simulink model "STEP2_W"  (Simulink 8.6)
settings: Solver=ode4  SolverMode=SingleTasking  StartTime=0.0  StopTime=inf  FixedStep=2/64e5  RelTol=1e-3
undefined symbols (not defined in the file or in its folder): get
libraries: system_blocks x3, measurement_tools x2, dspsnks4 x1
settings Model: MAModelExclusionFileProxy=C:\Users\user\Desktop\HAW\Digital Communication Systems\labs\Matlab\STEP2_W_exclusions.xml  Creator=Schoenen  LastModifiedBy=user
settings DataIOCC: SaveOutput=off  SaveTime=off  SignalLoggingName=sigsOut
settings OptimizationCC: BooleanDataType=off  ExpressionDepthLimit=128
settings DebuggingCC: SaveWithParameterizedLinksMsg=none  SignalResolutionControl=TryResolveAllWithWarning  SolverPrmCheckMsg=none  MultiTaskDSMMsg=warning  MultiTaskCondExecSysMsg=none  FcnCallInpInsideContextMsg=EnableAllAsError  StateNameClashWarn=none
settings HardwareCC: TargetUnknown=on
settings CodeAppCC: IgnoreCustomStorageClasses=off
settings ConfigComp: CovSFcnEnable=off

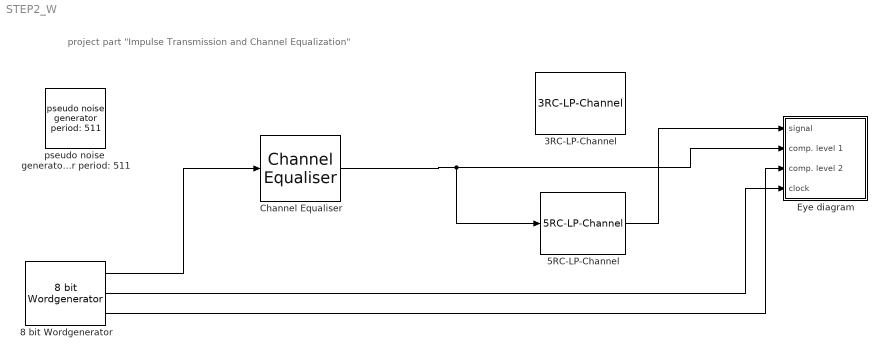
== system STEP2_W ==
  note: project part "Impulse Transmission and Channel Equalization"
  "3RC-LP-Channel " : system_blocks/3RC-LP-Channel   noise=0.1  a=off  step=2/64e5
  "5RC-LP-Channel " : system_blocks/5RC-LP-Channel   noise=0.1  a=off  step=2/64e5
  8 bit Wordgenerator : measurement_tools/8 bit Wordgenerator  word=[1 0 0 0 0 0 0 0]  bt=64000
  Channel Equaliser : system_blocks/Channel Equaliser
      link override c1: low=-1  gain=-0.733  high=1
      link override c2: low=-1  gain=0.227  high=1
      link override c3: low=-1  gain=-0.049  high=1
      link override c4: low=-1  gain=0.0026  high=1
  Eye diagram : Subsystem  AncestorBlock=measurement_tools/Eye diagram  mask{Tsymb=1, Tfss=2/64e5, ns=4, ndisplay=1, ymin=-2, ymax=2}
      mask prompts: Tsymb "symbol period [s]:"; Tfss "simulation step size [s]:"; ns "symbols per eye diagram (min. 4xndisplay):"; ndisplay "display time scale [ndisplay=number of symbols]:"
      mask init:
      | SampPerSymb = round(Tsymb/Tfss);
      | nsymb=ndisplay*ceil(ns/ndisplay);
  pseudo noise  generator period: 511 : measurement_tools/pseudo noise  generator period: 511  Tsymb=1  pol=unipolar  Tfss=2/64e5
  wires:
  8 bit Wordgenerator/3 -> Eye diagram/3(comp. level 2)
  8 bit Wordgenerator/2 -> Eye diagram/4(clock)
  8 bit Wordgenerator/1 -> Channel Equaliser/1
  Channel Equaliser/1 -> "5RC-LP-Channel "/1, Eye diagram/2(comp. level 1)
  "5RC-LP-Channel "/1 -> Eye diagram/1(signal)

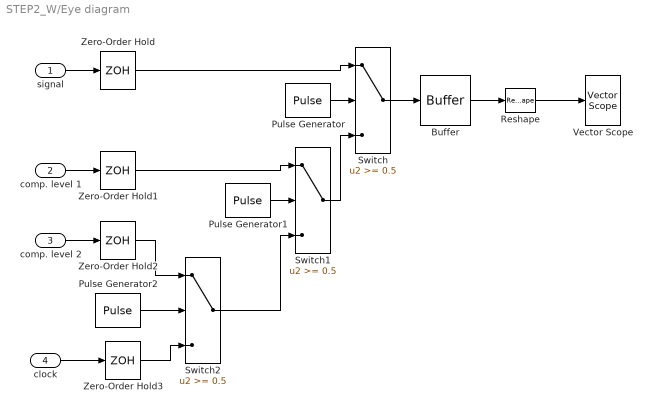
== system STEP2_W/Eye diagram ==
  signal : Inport
  comp. level 1 : Inport  Port=2
  comp. level 2 : Inport  Port=3
  clock : Inport  Port=4
  Buffer : Buffer  RequirementInfo="{}  %GIDa_20dddd1b_447a_4159_b5a4_549dd01b317e"  N=nsymb*SampPerSymb  TreatMby1Signals=One channel
  Pulse Generator : DiscretePulseGenerator  Period=nsymb*SampPerSymb  PulseWidth=(nsymb-3*ndisplay)*SampPerSymb  PhaseDelay=3*ndisplay*SampPerSymb  SampleTime=Tfss
  Pulse Generator1 : DiscretePulseGenerator  Period=nsymb*SampPerSymb  PulseWidth=ndisplay*SampPerSymb  SampleTime=Tfss
  Pulse Generator2 : DiscretePulseGenerator  Period=nsymb*SampPerSymb  PulseWidth=ndisplay*SampPerSymb  PhaseDelay=ndisplay*SampPerSymb  SampleTime=Tfss
  Reshape : Reshape  OutputDimensionality=Customize  OutputDimensions=[ndisplay*SampPerSymb,nsymb/ndisplay]
  Switch : Switch  Threshold=0.5  SaturateOnIntegerOverflow=on
  Switch1 : Switch  Threshold=0.5  SaturateOnIntegerOverflow=on
  Switch2 : Switch  Threshold=0.5  SaturateOnIntegerOverflow=on
  Vector Scope : dspsnks4/Vector Scope  ScopeProperties=off  Domain=Time  HorizSpan=1  DisplayProperties=off  AxisGrid=on  Memory=on  FrameNumber=on  AxisLegend=on  AxisZoom=off  OpenScopeAtSimStart=on  OpenScopeImmediately=off  FigPos=get(0,'defaultfigureposition')  AxisProperties=on  XUnits=Hertz  XRange=[0...Fs/2]  InheritXIncr=on  XIncr=1  XLabel=Time  XLimit=Auto  XMin=0  XMax=1  XStart=0  YUnits=dB  YLabel=Amplitude  LineProperties=off  LineDisables=on  LineStyles=-|-  LineColors=[1 0 0]|[0 1 0]|[0 0 1]  XAxisParamsVer=6.8
      settings: YMin=ymin  YMax=ymax
  Zero-Order Hold{,1..3} (4 alike) : ZeroOrderHold  SampleTime=Tfss
  wires:
  Buffer/1 -> Reshape/1
  Reshape/1 -> Vector Scope/1
  Zero-Order Hold/1 -> Switch/1
  Switch/1 -> Buffer/1
  Pulse Generator/1 -> Switch/2
  Zero-Order Hold1/1 -> Switch1/1
  Pulse Generator1/1 -> Switch1/2
  Switch1/1 -> Switch/3
  signal/1 -> Zero-Order Hold/1
  comp. level 1/1 -> Zero-Order Hold1/1
  comp. level 2/1 -> Zero-Order Hold2/1
  Zero-Order Hold2/1 -> Switch2/1
  clock/1 -> Zero-Order Hold3/1
  Zero-Order Hold3/1 -> Switch2/3
  Switch2/1 -> Switch1/3
  Pulse Generator2/1 -> Switch2/2
